simulink model "S2_ContinuousDCMotorSimulationFixPt2017a"  (Simulink 8.9)
settings: Solver=VariableStepAuto  StartTime=0.0  StopTime=25  MaxStep=Ts  RelTol=1e-3
undefined symbols (not defined in the file): C0, DiscIntNeverNeededParam, F, Imax, Imin, J, Ke, Km, Kphi, L, Ommax, Ommin, R, Ts, TsMeca, Vmax, Vmin
libraries: simulink x6
Description:
  | Continuous time model of the DC motor
  | 
  | Cascaded speed control :
  | - Inner loop : electrical control (state feedback with integral action)
  | - Outer loop :  mechanical control (state feedback with integral action)
  | - Clamping : Enable or disable integral actions
settings Model: Creator=R.Delpoux & L.Kerhuel  LastModifiedBy=rdelpoux
settings SolverCC: ZeroCrossControl=DisableAll
settings DataIOCC: LimitDataPoints=off  SaveFormat=Dataset  SignalLoggingSaveFormat=Dataset
settings OptimizationCC: LifeSpan=auto
settings DebuggingCC: UnderspecifiedInitializationDetection=Simplified  MergeDetectMultiDrivingBlocksExec=error  FcnCallInpInsideContextMsg=error  StateNameClashWarn=none  SFUnexpectedBacktrackingDiag=error  SFNoUnconditionalDefaultTransitionDiag=error  SFExecutionAtInitializationDiag=warning
settings HardwareCC: ProdBitPerPointer=64  ProdBitPerSizeT=64  ProdBitPerPtrDiffT=64  ProdLargestAtomicFloat=Float  ProdIntDivRoundTo=Zero  ProdEndianess=LittleEndian  ProdWordSize=64  ProdHWDeviceType=Intel->x86-64 (Windows64)
settings ModelReferenceCC: PropagateSignalLabelsOutOfModel=on
settings GRTTargetCC: TargetLangStandard=C99 (ISO)  GeneratePreprocessorConditionals=Use local settings  CombineOutputUpdateFcns=on  GRTInterface=off
settings ConfigComp: CovMetricSettings=dwe  CovHtmlReporting=off  CovSaveCumulativeToWorkspaceVar=off  CovSaveSingleToWorkspaceVar=off  CovExternalEMLEnable=on

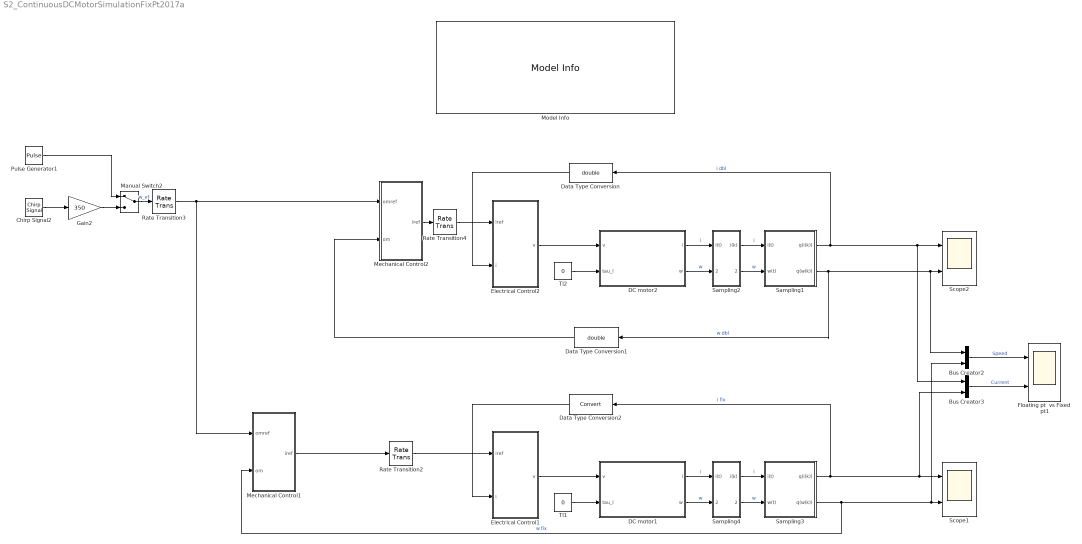
== system S2_ContinuousDCMotorSimulationFixPt2017a ==
  Bus Creator2 : BusCreator  Inputs=2
  Bus Creator3 : BusCreator  Inputs=2
  Chirp Signal2 : simulink/Sources/Chirp Signal  f1=0.1  T=20  f2=5
  DC motor1 : Subsystem  mask(Motor PRAVALUX MPM4-0002){R=R, L=L, Kphi=Kphi, J=J, F=F, C0=C0}
      mask prompts: R "Resistance (R) in Ohms"; L "Inductance (L) in H"; Kphi "Back EMF (Kphi) in V/rad/s"; J "J in kgm²"; F "F in N/rad/s"
      mask help:
      | Continuous time Model for PRAVALUX MPM4 DC motor
      | Caracteristics: 24V DC, 90W, 5.2A, 3000RPM
      |
      | It is a 2nd order model made of two intertwinned system:
      | one 1st order electrical system and one 1st order mechanical system.
      |
      | Look under mask (Ctrl-U) to see the model
      mask DialogControl Container11 Prompt: Motor
      mask Display:
      | color('green');
      | image('MotorPravalux.png');
      | %port_label('input',1,'DC');
      | %port_label('output',1,'BEMF');
  DC motor2 : Subsystem  mask(Motor PRAVALUX MPM4-0002){R=R, L=L, Kphi=Kphi, J=J, F=F, C0=C0}
      mask prompts: R "Resistance (R) in Ohms"; L "Inductance (L) in H"; Kphi "Back EMF (Kphi) in V/rad/s"; J "J in kgm²"; F "F in N/rad/s"
      mask help:
      | Continuous time Model for PRAVALUX MPM4 DC motor
      | Caracteristics: 24V DC, 90W, 5.2A, 3000RPM
      |
      | It is a 2nd order model made of two intertwinned system:
      | one 1st order electrical system and one 1st order mechanical system.
      |
      | Look under mask (Ctrl-U) to see the model
      mask DialogControl Container11 Prompt: Motor
      mask Display:
      | color('green');
      | image('MotorPravalux.png');
      | %port_label('input',1,'DC');
      | %port_label('output',1,'BEMF');
  Data Type Conversion : DataTypeConversion  OutDataTypeStr=double
  Data Type Conversion1 : DataTypeConversion  OutDataTypeStr=double
  Data Type Conversion2 : DataTypeConversion
  Electrical Control1 : Subsystem
  Electrical Control2 : Subsystem
  Floating pt  vs Fixed pt1 : Scope  NumInputPorts=2
  Gain2 : Gain  Gain=350  OutDataTypeStr=Inherit: Inherit via back propagation
  Manual Switch2 : ManualSwitch
  Mechanical Control1 : Subsystem
  Mechanical Control2 : Subsystem
  Model Info : simulink/Model-Wide Utilities/Model Info  Frame=on  DisplayStringWithTags=|  HorizontalTextAlignment=Center  LeftAlignmentValue=0.5
      | %<ModelName> v%<ModelVersion> - %<Creator>
      | 
      | %<Description>
      | 
      | Lost modified on: %<LastModificationDate>
  Pulse Generator1 : DiscretePulseGenerator  PulseType=Time based  Amplitude=200  PulseWidth=50  PhaseDelay=0.5  SampleTime=-1
  Rate Transition2 : RateTransition  Deterministic=off
  Rate Transition3 : RateTransition  Deterministic=off
  Rate Transition4 : RateTransition  Deterministic=off
  Sampling1 : Subsystem
  Sampling2 : Subsystem
  Sampling3 : Subsystem
  Sampling4 : Subsystem
  Scope1 : Scope  NumInputPorts=2
  Scope2 : Scope  NumInputPorts=2
  Tl1 : Constant  Value=0
  Tl2 : Constant  Value=0
  wires:
  Mechanical Control2/1(iref) -> Rate Transition4/1
  DC motor2/2(w) -> Sampling2/2(w(t))  "w"
  DC motor2/1(i) -> Sampling2/1(i(t))  "i"
  Manual Switch2/1 -> Rate Transition3/1  "w_ef"
  Chirp Signal2/1 -> Gain2/1
  Gain2/1 -> Manual Switch2/2
  Tl2/1 -> DC motor2/2(tau_l)
  Electrical Control2/1(v) -> DC motor2/1(v)
  Pulse Generator1/1 -> Manual Switch2/1
  Sampling1/1(q(i(k))) -> Bus Creator3/1, Scope2/1, Data Type Conversion/1  "i dbl"
  Sampling1/2(q(w(k))) -> Bus Creator2/1, Scope2/2, Data Type Conversion1/1  "w dbl"
  Sampling2/1(i(k)) -> Sampling1/1(i(t))  "i"
  Sampling2/2(w(k)) -> Sampling1/2(w(t))  "w"
  Data Type Conversion/1 -> Electrical Control2/2(i)
  Data Type Conversion1/1 -> Mechanical Control2/2(om)
  Rate Transition4/1 -> Electrical Control2/1(iref)
  Rate Transition2/1 -> Electrical Control1/1(iref)
  Rate Transition3/1 -> Mechanical Control1/1(omref), Mechanical Control2/1(omref)
  Data Type Conversion2/1 -> Electrical Control1/2(i)
  Sampling4/2(w(k)) -> Sampling3/2(w(t))  "w"
  Sampling4/1(i(k)) -> Sampling3/1(i(t))  "i"
  Sampling3/2(q(w(k))) -> Mechanical Control1/2(om), Bus Creator2/2, Scope1/2  "w fix"
  Sampling3/1(q(i(k))) -> Data Type Conversion2/1, Bus Creator3/2, Scope1/1  "i fix"
  Electrical Control1/1(v) -> DC motor1/1(v)
  Tl1/1 -> DC motor1/2(tau_l)
  DC motor1/1(i) -> Sampling4/1(i(t))  "i"
  DC motor1/2(w) -> Sampling4/2(w(t))  "w"
  Mechanical Control1/1(iref) -> Rate Transition2/1
  Bus Creator3/1 -> Floating pt  vs Fixed pt1/2  "Current"
  Bus Creator2/1 -> Floating pt  vs Fixed pt1/1  "Speed"

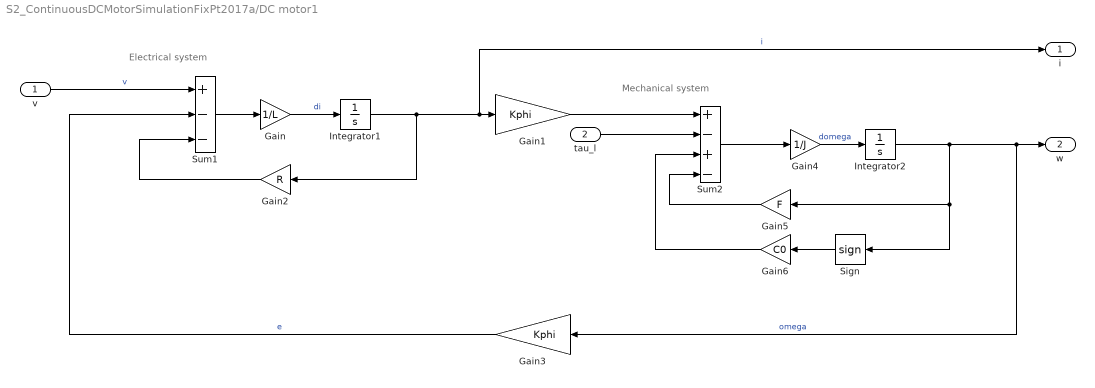
== system S2_ContinuousDCMotorSimulationFixPt2017a/DC motor1 ==
  note: Mechanical system
  note: Electrical system
  v : Inport  SampleTime=0
  tau_l : Inport  Port=2
  Gain : Gain  Gain=1/L
  Gain1 : Gain  Gain=Kphi
  Gain2 : Gain  Gain=R
  "Gain3  " : Gain  Gain=Kphi
  Gain4 : Gain  Gain=1/J
  Gain5 : Gain  Gain=F
  Gain6 : Gain  Gain=C0
  Integrator1 : Integrator
  Integrator2 : Integrator
  Sign : Signum
  Sum1 : Sum  Inputs=+--
  Sum2 : Sum  Inputs=+-+-
  i : Outport
  w : Outport  Port=2
  wires:
  Sum1/1 -> Gain/1
  Gain/1 -> Integrator1/1  "di"
  Integrator1/1 -> Gain2/1, i/1, Gain1/1  "i"
  v/1 -> Sum1/1  "v"
  Gain2/1 -> Sum1/3
  "Gain3  "/1 -> Sum1/2  "e"
  tau_l/1 -> Sum2/2
  Gain6/1 -> Sum2/3
  Sign/1 -> Gain6/1
  Integrator2/1 -> "Gain3  "/1, w/1, Sign/1, Gain5/1  "omega"
  Gain5/1 -> Sum2/4
  Sum2/1 -> Gain4/1
  Gain4/1 -> Integrator2/1  "domega"
  Gain1/1 -> Sum2/1

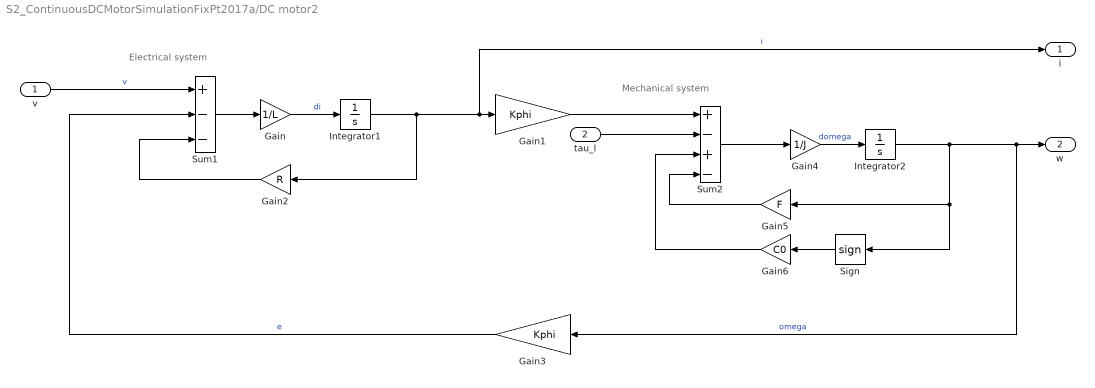
== system S2_ContinuousDCMotorSimulationFixPt2017a/DC motor2 ==
  note: Electrical system
  note: Mechanical system
  v : Inport  SampleTime=0
  tau_l : Inport  Port=2
  Gain : Gain  Gain=1/L
  Gain1 : Gain  Gain=Kphi
  Gain2 : Gain  Gain=R
  "Gain3  " : Gain  Gain=Kphi
  Gain4 : Gain  Gain=1/J
  Gain5 : Gain  Gain=F
  Gain6 : Gain  Gain=C0
  Integrator1 : Integrator
  Integrator2 : Integrator
  Sign : Signum
  Sum1 : Sum  Inputs=+--
  Sum2 : Sum  Inputs=+-+-
  i : Outport
  w : Outport  Port=2
  wires:
  Gain1/1 -> Sum2/1
  Gain4/1 -> Integrator2/1  "domega"
  Sum2/1 -> Gain4/1
  Gain5/1 -> Sum2/4
  Integrator2/1 -> Gain5/1, Sign/1, w/1, "Gain3  "/1  "omega"
  Sign/1 -> Gain6/1
  Gain6/1 -> Sum2/3
  tau_l/1 -> Sum2/2
  "Gain3  "/1 -> Sum1/2  "e"
  Gain2/1 -> Sum1/3
  v/1 -> Sum1/1  "v"
  Integrator1/1 -> Gain1/1, i/1, Gain2/1  "i"
  Gain/1 -> Integrator1/1  "di"
  Sum1/1 -> Gain/1

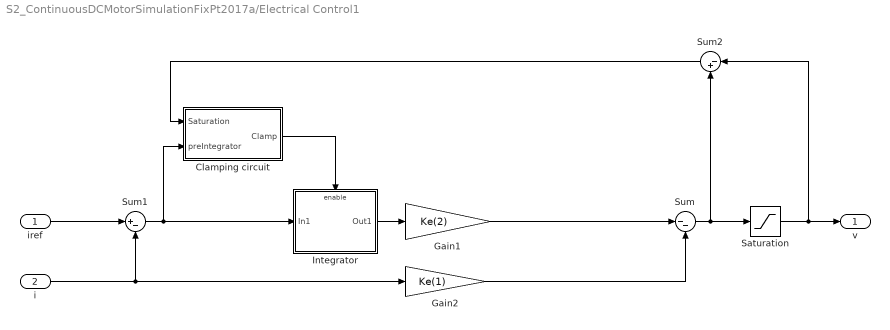
== system S2_ContinuousDCMotorSimulationFixPt2017a/Electrical Control1 ==
  iref : Inport
  i : Inport  Port=2
  Clamping circuit : Subsystem
  Gain1 : Gain  Gain=Ke(2)  OutMin=[2*Vmin]  OutMax=[2*Vmax]  OutDataTypeStr=fixdt(1,16)
  Gain2 : Gain  Gain=Ke(1)  OutMin=[2*Vmin]  OutMax=[2*Vmax]  OutDataTypeStr=fixdt(1,16)
  Integrator : Subsystem
  Saturation : Saturate  UpperLimit=Vmax  LowerLimit=Vmin
  Sum : Sum  Inputs=|--
  Sum1 : Sum  Inputs=|+-  OutMin=[2*Imin]  OutMax=[2*Imax]  OutDataTypeStr=fixdt(1,16)
  Sum2 : Sum  Inputs=|-+  OutDataTypeStr=Inherit: Same as accumulator
  v : Outport
  wires:
  iref/1 -> Sum1/1
  i/1 -> Gain2/1, Sum1/2
  Gain1/1 -> Sum/1
  Gain2/1 -> Sum/2
  Saturation/1 -> Sum2/1, v/1
  Sum1/1 -> Integrator/1(In1), Clamping circuit/2(preIntegrator)
  Integrator/1(Out1) -> Gain1/1
  Clamping circuit/1(Clamp) -> Integrator/Enable
  Sum/1 -> Saturation/1, Sum2/2
  Sum2/1 -> Clamping circuit/1(Saturation)

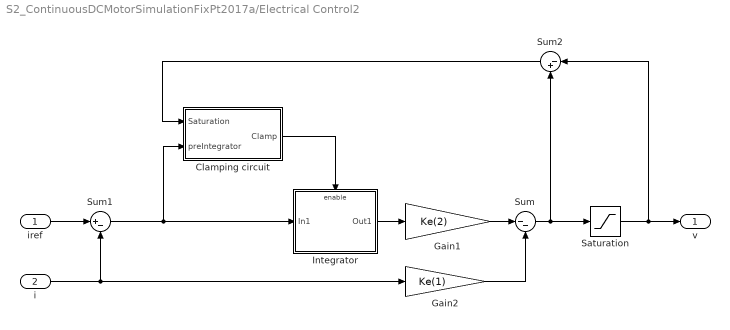
== system S2_ContinuousDCMotorSimulationFixPt2017a/Electrical Control2 ==
  iref : Inport
  i : Inport  Port=2
  Clamping circuit : Subsystem
  Gain1 : Gain  Gain=Ke(2)
  Gain2 : Gain  Gain=Ke(1)
  Integrator : Subsystem
  Saturation : Saturate  UpperLimit=Vmax  LowerLimit=Vmin
  Sum : Sum  Inputs=|--
  Sum1 : Sum  Inputs=|+-
  Sum2 : Sum  Inputs=|-+  OutDataTypeStr=Inherit: Same as accumulator
  v : Outport
  wires:
  Sum2/1 -> Clamping circuit/1(Saturation)
  Sum/1 -> Sum2/2, Saturation/1
  Clamping circuit/1(Clamp) -> Integrator/Enable
  Integrator/1(Out1) -> Gain1/1
  Sum1/1 -> Clamping circuit/2(preIntegrator), Integrator/1(In1)
  Saturation/1 -> v/1, Sum2/1
  Gain2/1 -> Sum/2
  Gain1/1 -> Sum/1
  i/1 -> Sum1/2, Gain2/1
  iref/1 -> Sum1/1

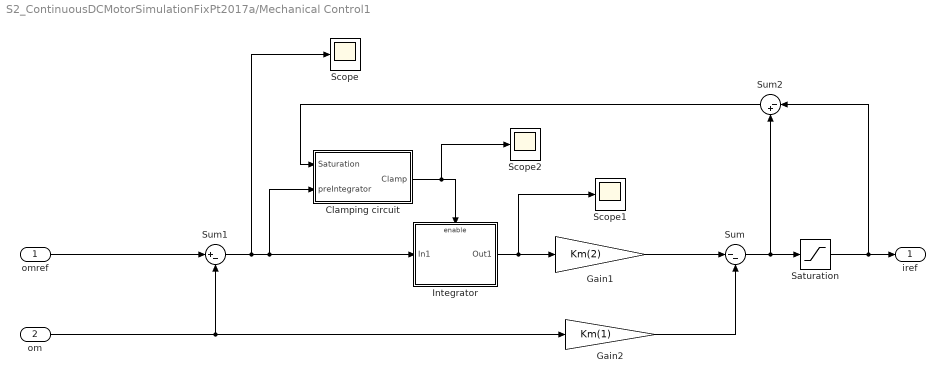
== system S2_ContinuousDCMotorSimulationFixPt2017a/Mechanical Control1 ==
  omref : Inport  OutMin=[Ommin]  OutMax=[Ommax]  OutDataTypeStr=fixdt(1,16)
  om : Inport  Port=2
  Clamping circuit : Subsystem
  Gain1 : Gain  Gain=Km(2)  OutMin=[-2*Imax]  OutMax=[2*Imax]  OutDataTypeStr=fixdt(1,16)
  Gain2 : Gain  Gain=Km(1)  OutMin=[-2*Imax]  OutMax=[2*Imax]  OutDataTypeStr=fixdt(1,16)
  Integrator : Subsystem
  Saturation : Saturate  UpperLimit=Imax  LowerLimit=Imin
  Scope : Scope
  Scope1 : Scope
  Scope2 : Scope
  Sum : Sum  Inputs=|--
  Sum1 : Sum  Inputs=|+-  OutMin=[2*Ommin]  OutMax=[2*Ommax]  OutDataTypeStr=fixdt(1,16)
  Sum2 : Sum  Inputs=|-+  OutDataTypeStr=Inherit: Same as accumulator
  iref : Outport
  wires:
  Gain1/1 -> Sum/1
  Sum1/1 -> Scope/1, Clamping circuit/2(preIntegrator), Integrator/1(In1)
  omref/1 -> Sum1/1
  Gain2/1 -> Sum/2
  om/1 -> Gain2/1, Sum1/2
  Sum2/1 -> Clamping circuit/1(Saturation)
  Sum/1 -> Sum2/2, Saturation/1
  Clamping circuit/1(Clamp) -> Scope2/1, Integrator/Enable
  Saturation/1 -> Sum2/1, iref/1
  Integrator/1(Out1) -> Scope1/1, Gain1/1

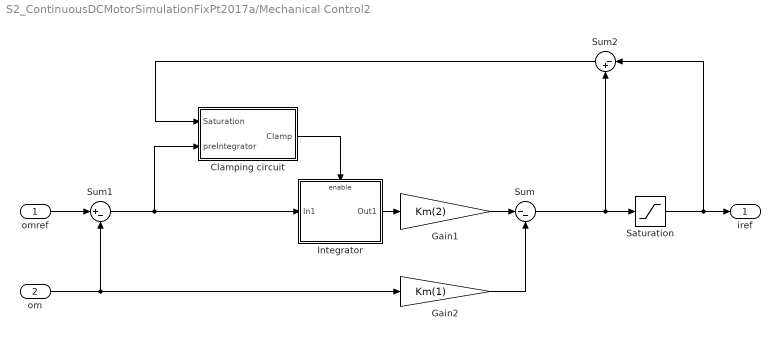
== system S2_ContinuousDCMotorSimulationFixPt2017a/Mechanical Control2 ==
  omref : Inport
  om : Inport  Port=2
  Clamping circuit : Subsystem
  Gain1 : Gain  Gain=Km(2)
  Gain2 : Gain  Gain=Km(1)
  Integrator : Subsystem
  Saturation : Saturate  UpperLimit=Imax  LowerLimit=Imin
  Sum : Sum  Inputs=|--
  Sum1 : Sum  Inputs=|+-
  Sum2 : Sum  Inputs=|-+  OutDataTypeStr=Inherit: Same as accumulator
  iref : Outport
  wires:
  Integrator/1(Out1) -> Gain1/1
  Saturation/1 -> iref/1, Sum2/1
  Clamping circuit/1(Clamp) -> Integrator/Enable
  Sum/1 -> Saturation/1, Sum2/2
  Sum2/1 -> Clamping circuit/1(Saturation)
  om/1 -> Sum1/2, Gain2/1
  Gain2/1 -> Sum/2
  omref/1 -> Sum1/1
  Sum1/1 -> Integrator/1(In1), Clamping circuit/2(preIntegrator)
  Gain1/1 -> Sum/1

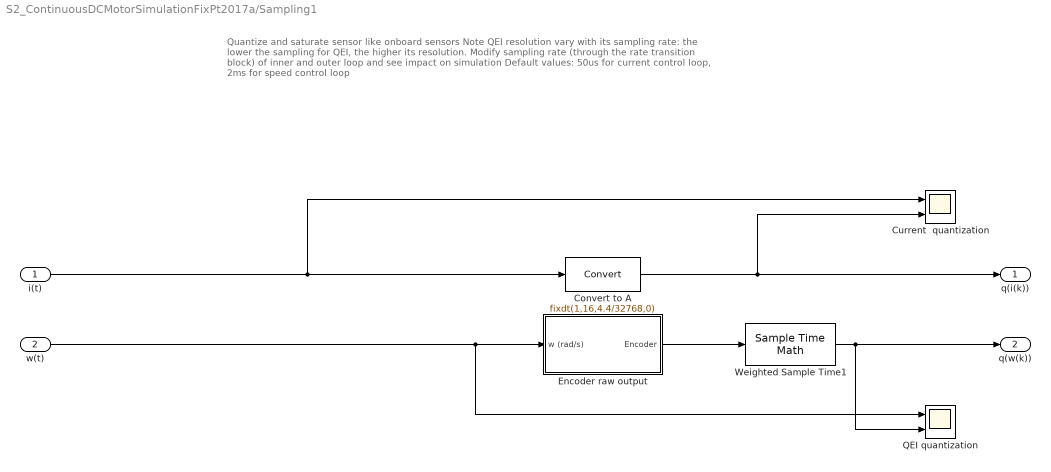
== system S2_ContinuousDCMotorSimulationFixPt2017a/Sampling1 ==
  note: Quantize and saturate sensor like onboard sensors
      |
      | Note QEI resolution vary with its sampling rate:
      | the lower the sampling for QEI, the higher its resolution.
      |
      | Modify sampling rate (through the rate transition block) of inner and outer loop and see impact on simulation
      |
      | Default values: 50us for current control loop, 2ms for speed control loop
  i(t) : Inport
  w(t) : Inport  Port=2
  Convert to A : DataTypeConversion  OutDataTypeStr=fixdt(1,16,4.4/32768,0)  SaturateOnIntegerOverflow=on  LockScale=on
  Current  quantization : Scope  NumInputPorts=2
  Encoder raw output : Subsystem
  QEI quantization : Scope  NumInputPorts=2
  Weighted Sample Time1 : SampleTimeMath  TsampMathOp=/  weightValue=1000/pi  TsampMathImp=Offline Scaling Adjustment
  q(i(k)) : Outport
  q(w(k)) : Outport  Port=2
  wires:
  w(t)/1 -> QEI quantization/1, Encoder raw output/1(w (rad/s))
  Weighted Sample Time1/1 -> QEI quantization/2, q(w(k))/1
  Encoder raw output/1(Encoder) -> Weighted Sample Time1/1
  Convert to A/1 -> q(i(k))/1, Current  quantization/2
  i(t)/1 -> Convert to A/1, Current  quantization/1

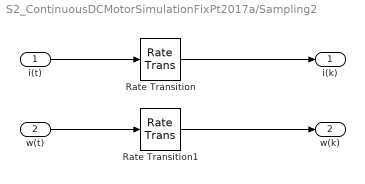
== system S2_ContinuousDCMotorSimulationFixPt2017a/Sampling2 ==
  i(t) : Inport
  w(t) : Inport  Port=2
  Rate Transition : RateTransition  Deterministic=off  OutPortSampleTime=Ts
  Rate Transition1 : RateTransition  Deterministic=off  OutPortSampleTime=TsMeca
  i(k) : Outport
  w(k) : Outport  Port=2
  wires:
  Rate Transition1/1 -> w(k)/1
  w(t)/1 -> Rate Transition1/1
  i(t)/1 -> Rate Transition/1
  Rate Transition/1 -> i(k)/1

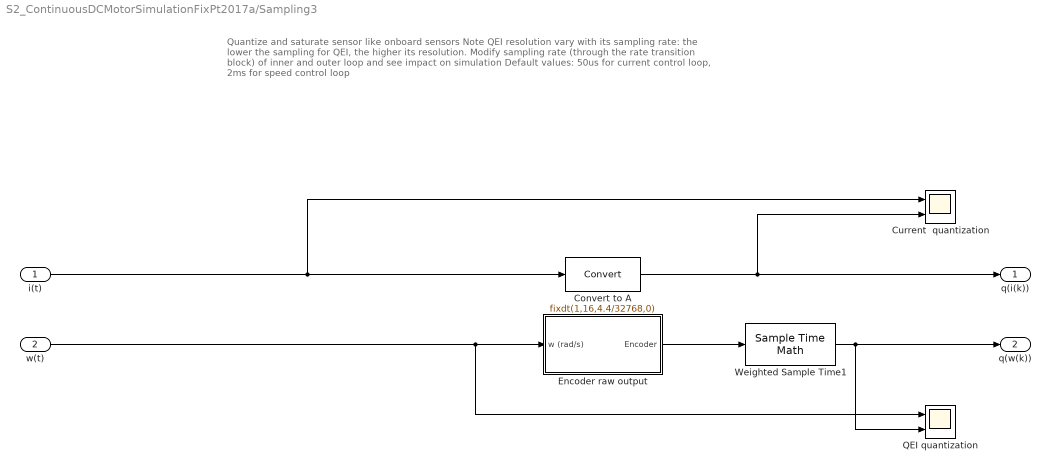
== system S2_ContinuousDCMotorSimulationFixPt2017a/Sampling3 ==
  note: Quantize and saturate sensor like onboard sensors
      |
      | Note QEI resolution vary with its sampling rate:
      | the lower the sampling for QEI, the higher its resolution.
      |
      | Modify sampling rate (through the rate transition block) of inner and outer loop and see impact on simulation
      |
      | Default values: 50us for current control loop, 2ms for speed control loop
  i(t) : Inport
  w(t) : Inport  Port=2
  Convert to A : DataTypeConversion  OutDataTypeStr=fixdt(1,16,4.4/32768,0)  SaturateOnIntegerOverflow=on  LockScale=on
  Current  quantization : Scope  NumInputPorts=2
  Encoder raw output : Subsystem
  QEI quantization : Scope  NumInputPorts=2
  Weighted Sample Time1 : SampleTimeMath  TsampMathOp=/  weightValue=1000/pi  TsampMathImp=Offline Scaling Adjustment
  q(i(k)) : Outport
  q(w(k)) : Outport  Port=2
  wires:
  i(t)/1 -> Current  quantization/1, Convert to A/1
  Convert to A/1 -> Current  quantization/2, q(i(k))/1
  Encoder raw output/1(Encoder) -> Weighted Sample Time1/1
  Weighted Sample Time1/1 -> q(w(k))/1, QEI quantization/2
  w(t)/1 -> Encoder raw output/1(w (rad/s)), QEI quantization/1

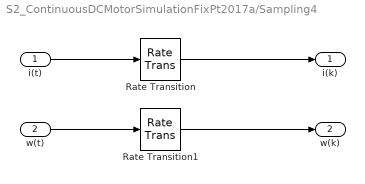
== system S2_ContinuousDCMotorSimulationFixPt2017a/Sampling4 ==
  i(t) : Inport
  w(t) : Inport  Port=2
  Rate Transition : RateTransition  Deterministic=off  OutPortSampleTime=Ts
  Rate Transition1 : RateTransition  Deterministic=off  OutPortSampleTime=TsMeca
  i(k) : Outport
  w(k) : Outport  Port=2
  wires:
  Rate Transition/1 -> i(k)/1
  i(t)/1 -> Rate Transition/1
  w(t)/1 -> Rate Transition1/1
  Rate Transition1/1 -> w(k)/1

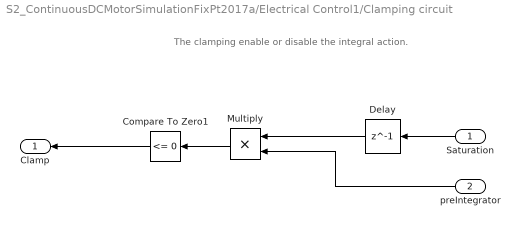
== system S2_ContinuousDCMotorSimulationFixPt2017a/Electrical Control1/Clamping circuit ==
  note: The clamping enable or disable the integral action.
  Saturation : Inport  DisableCoverage=on
  preIntegrator : Inport  DisableCoverage=on  Port=2
  Compare To Zero1 : simulink/Logic and Bit Operations/Compare To Zero  relop=<=  OutDataTypeStr=boolean
  Delay : Delay  DelayLength=1  InitialCondition=0
  Multiply : Product
  Clamp : Outport  DisableCoverage=on
  wires:
  Compare To Zero1/1 -> Clamp/1
  preIntegrator/1 -> Multiply/2
  Multiply/1 -> Compare To Zero1/1
  Saturation/1 -> Delay/1
  Delay/1 -> Multiply/1

== system S2_ContinuousDCMotorSimulationFixPt2017a/Electrical Control1/Integrator ==
  In1 : Inport
  Enable : EnablePort
  Discrete-Time Integrator : DiscreteIntegrator  InitialConditionSetting=State (most efficient)  SampleTime=Ts  OutMin=[2*Imin]  OutMax=[2*Imax]  OutDataTypeStr=fixdt(1,32)  ICPrevOutput=DiscIntNeverNeededParam  ICPrevScaledInput=DiscIntNeverNeededParam
  Out1 : Outport
  wires:
  Discrete-Time Integrator/1 -> Out1/1
  In1/1 -> Discrete-Time Integrator/1

== system S2_ContinuousDCMotorSimulationFixPt2017a/Electrical Control2/Clamping circuit ==
  note: The clamping enable or disable the integral action.
  Saturation : Inport  DisableCoverage=on
  preIntegrator : Inport  DisableCoverage=on  Port=2
  Compare To Zero1 : simulink/Logic and Bit Operations/Compare To Zero  relop=<=  OutDataTypeStr=boolean
  Delay : Delay  DelayLength=1  InitialCondition=0
  Multiply : Product
  Clamp : Outport  DisableCoverage=on
  wires:
  Delay/1 -> Multiply/1
  Saturation/1 -> Delay/1
  Multiply/1 -> Compare To Zero1/1
  preIntegrator/1 -> Multiply/2
  Compare To Zero1/1 -> Clamp/1

== system S2_ContinuousDCMotorSimulationFixPt2017a/Electrical Control2/Integrator ==
  In1 : Inport
  Enable : EnablePort
  Discrete-Time Integrator : DiscreteIntegrator  InitialConditionSetting=State (most efficient)  SampleTime=Ts  ICPrevOutput=DiscIntNeverNeededParam  ICPrevScaledInput=DiscIntNeverNeededParam
  Out1 : Outport
  wires:
  In1/1 -> Discrete-Time Integrator/1
  Discrete-Time Integrator/1 -> Out1/1

== system S2_ContinuousDCMotorSimulationFixPt2017a/Mechanical Control1/Clamping circuit ==
  note: La logique de clamping permet de bloquer l'entée de l'action intégrale.
      | Ainsi, si la sortie du controlleur est en dehors des limites imposés (saturée), alors l'action intégrale du correcteur est verrouyé (clamping).
      | L'action intégrale est verroullé si la sortie du correcteur (commande) est en dehors des saturations et que le signe de cette sortie est égale
      | à l'entrée du signal à intégrer.
  Saturation : Inport  DisableCoverage=on
  preIntegrator : Inport  DisableCoverage=on  Port=2
  Compare To Zero1 : simulink/Logic and Bit Operations/Compare To Zero  relop=<=  OutDataTypeStr=boolean
  Delay : Delay  DelayLength=1  InitialCondition=0  SampleTime=TsMeca
  Multiply : Product
  Clamp : Outport  DisableCoverage=on
  wires:
  Compare To Zero1/1 -> Clamp/1
  preIntegrator/1 -> Multiply/2
  Multiply/1 -> Compare To Zero1/1
  Saturation/1 -> Delay/1
  Delay/1 -> Multiply/1

== system S2_ContinuousDCMotorSimulationFixPt2017a/Mechanical Control1/Integrator ==
  In1 : Inport
  Enable : EnablePort
  Discrete-Time Integrator : DiscreteIntegrator  InitialConditionSetting=State (most efficient)  SampleTime=TsMeca  OutMin=[2*Ommin]  OutMax=[2*Ommax]  OutDataTypeStr=fixdt(1,32)  ICPrevOutput=DiscIntNeverNeededParam  ICPrevScaledInput=DiscIntNeverNeededParam
  Out1 : Outport
  wires:
  Discrete-Time Integrator/1 -> Out1/1
  In1/1 -> Discrete-Time Integrator/1

== system S2_ContinuousDCMotorSimulationFixPt2017a/Mechanical Control2/Clamping circuit ==
  note: La logique de clamping permet de bloquer l'entée de l'action intégrale.
      | Ainsi, si la sortie du controlleur est en dehors des limites imposés (saturée), alors l'action intégrale du correcteur est verrouyé (clamping).
      | L'action intégrale est verroullé si la sortie du correcteur (commande) est en dehors des saturations et que le signe de cette sortie est égale
      | à l'entrée du signal à intégrer.
  Saturation : Inport  DisableCoverage=on
  preIntegrator : Inport  DisableCoverage=on  Port=2
  Compare To Zero1 : simulink/Logic and Bit Operations/Compare To Zero  relop=<=  OutDataTypeStr=boolean
  Delay : Delay  DelayLength=1  InitialCondition=0  SampleTime=TsMeca
  Multiply : Product
  Clamp : Outport  DisableCoverage=on
  wires:
  Delay/1 -> Multiply/1
  Saturation/1 -> Delay/1
  Multiply/1 -> Compare To Zero1/1
  preIntegrator/1 -> Multiply/2
  Compare To Zero1/1 -> Clamp/1

== system S2_ContinuousDCMotorSimulationFixPt2017a/Mechanical Control2/Integrator ==
  In1 : Inport
  Enable : EnablePort
  Discrete-Time Integrator : DiscreteIntegrator  InitialConditionSetting=State (most efficient)  SampleTime=TsMeca  ICPrevOutput=DiscIntNeverNeededParam  ICPrevScaledInput=DiscIntNeverNeededParam
  Out1 : Outport
  wires:
  In1/1 -> Discrete-Time Integrator/1
  Discrete-Time Integrator/1 -> Out1/1

== system S2_ContinuousDCMotorSimulationFixPt2017a/Sampling1/Encoder raw output ==
  w (rad/s) : Inport
  Encoder output : DataTypeConversion  OutDataTypeStr=int16  SaturateOnIntegerOverflow=on  LockScale=on
  Weighted Sample Time1 : SampleTimeMath  TsampMathOp=*  weightValue=1000/pi
  Encoder : Outport
  wires:
  w (rad/s)/1 -> Weighted Sample Time1/1
  Encoder output/1 -> Encoder/1
  Weighted Sample Time1/1 -> Encoder output/1

== system S2_ContinuousDCMotorSimulationFixPt2017a/Sampling3/Encoder raw output ==
  w (rad/s) : Inport
  Encoder output : DataTypeConversion  OutDataTypeStr=int16  SaturateOnIntegerOverflow=on  LockScale=on
  Weighted Sample Time1 : SampleTimeMath  TsampMathOp=*  weightValue=1000/pi
  Encoder : Outport
  wires:
  Weighted Sample Time1/1 -> Encoder output/1
  Encoder output/1 -> Encoder/1
  w (rad/s)/1 -> Weighted Sample Time1/1
